simulink model "simu7"  (R2018b)
settings: Solver=VariableStepAuto  StartTime=0.0  StopTime=100.0  RelTol=1e-3
values from neighbouring files (symbols this model uses):
  A1 = k(1)    [Lab6.m]    (also in script7.m = 1; test.m)
  A2 = k(1)    [Lab6.m]    (also in script7.m = 1; test.m)
  Aw1 = 0.1 * k(1)    [Lab6.m]    (also in script7.m = 0.1; test.m)
  Aw2 = 0.1 * k(1)    [Lab6.m]    (also in script7.m = 0.2; test.m)
  dfwe1 = 0    [script7.m]    (also in test.m = 0.2 * fwe1max)
  dfwe2 = 0    [script7.m]    (also in test.m = 0.1 * fwe2max)
  dt = 20    [script7.m]    (also in test.m)
  fwe1 = fwe10    [script7.m]    (also in test.m = fwe10(i))
  fwe2 = fwe20    (= 0)    [script7.m]    (also in test.m = fwe20(i))
  g = 9.81    [Lab6.m]    (also in script7.m; test.m)
  h10 = (fwe1 * fwe1)/(2 * g * Aw1 * Aw1) + h20    [script7.m]    (also in test.m = fwe1^2/(2*Aw1^2*g) + h20)
  h20 = 1/(2 * g * Aw2 * Aw2) * (fwe1 - fwe2) * (fwe1 - fwe2)    [script7.m]    (also in test.m = ((fwe1 + fwe2)^2) / (2*(Aw2^2)*g))
settings Model: Creator=wojciechkonury  LastModifiedBy=wojciechkonury

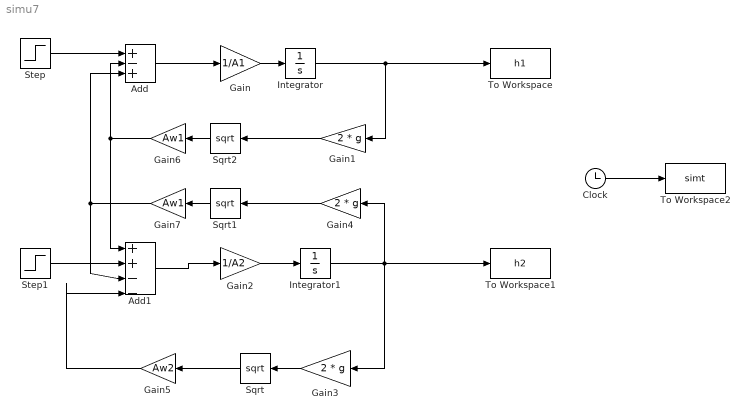
== system simu7 ==
  Add : Sum  Inputs=+-+
  Add1 : Sum  Inputs=+|+|-|-
  Clock : Clock
  Gain : Gain  Gain=1/A1
  Gain1 : Gain  Gain=2 * g
  Gain2 : Gain  Gain=1/A2
  Gain3 : Gain  Gain=2 * g
  Gain4 : Gain  Gain=2 * g
  Gain5 : Gain  Gain=Aw2
  Gain6 : Gain  Gain=Aw1
  Gain7 : Gain  Gain=Aw1
  Integrator : Integrator  InitialCondition=h10
  Integrator1 : Integrator  InitialCondition=h20
  Sqrt : Sqrt  IntermediateResultsDataTypeStr=double  SaturateOnIntegerOverflow=on
  Sqrt1 : Sqrt  IntermediateResultsDataTypeStr=double  SaturateOnIntegerOverflow=on
  Sqrt2 : Sqrt  IntermediateResultsDataTypeStr=double  SaturateOnIntegerOverflow=on
  Step : Step  Time=dt  Before=fwe1  After=fwe1+dfwe1  SampleTime=0
  Step1 : Step  Time=dt  Before=fwe2  After=fwe2+dfwe2  SampleTime=0
  To Workspace : ToWorkspace  VariableName=h1  SampleTime=-1
  To Workspace1 : ToWorkspace  VariableName=h2  SampleTime=-1
  To Workspace2 : ToWorkspace  VariableName=simt  SampleTime=-1
  wires:
  Step/1 -> Add/1
  Add/1 -> Gain/1
  Gain/1 -> Integrator/1
  Step1/1 -> Add1/2
  Integrator/1 -> Gain1/1, To Workspace/1
  Gain1/1 -> Sqrt2/1
  Add1/1 -> Gain2/1
  Gain2/1 -> Integrator1/1
  Integrator1/1 -> Gain4/1, To Workspace1/1, Gain3/1
  Gain3/1 -> Sqrt/1
  Gain4/1 -> Sqrt1/1
  Clock/1 -> To Workspace2/1
  Sqrt/1 -> Gain5/1
  Sqrt2/1 -> Gain6/1
  Sqrt1/1 -> Gain7/1
  Gain5/1 -> Add1/4
  Gain6/1 -> Add1/1, Add/2
  Gain7/1 -> Add1/3, Add/3
